simulink model "P01"  (R2019b)
settings: Solver=VariableStepAuto  StartTime=0.0  StopTime=200.0  RelTol=1e-3
settings Model: Creator=Alumno  LastModifiedBy=jpramez

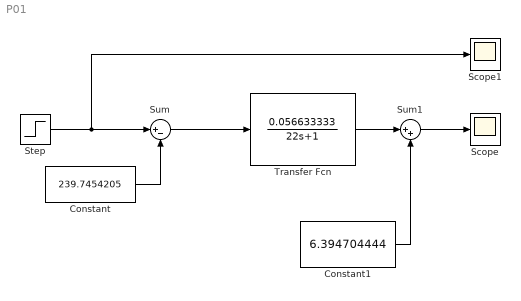
== system P01 ==
  Constant : Constant  Value=239.7454205
  Constant1 : Constant  Value=6.394704444
  Scope : Scope
  Scope1 : Scope
  Step : Step  Time=3  Before=239.7454205  After=239.7454205+30  SampleTime=0
  Sum : Sum  Inputs=|+-
  Sum1 : Sum  Inputs=|++
  Transfer Fcn : TransferFcn  Numerator=[0.056633333]  Denominator=[22 1]
  wires:
  Step/1 -> Sum/1, Scope1/1
  Sum/1 -> Transfer Fcn/1
  Constant/1 -> Sum/2
  Transfer Fcn/1 -> Sum1/1
  Sum1/1 -> Scope/1
  Constant1/1 -> Sum1/2
